simulink model "differential_steer"  (R2017b)
settings: Solver=FixedStepAuto  StartTime=0.0  StopTime=5  FixedStep=0.002  RelTol=1e-3
values from neighbouring files (symbols this model uses):
  B = 0.5    [main_differential_steer.m]
  input_type = 3    [main_bicycle.m]    (also in main_differential_steer.m; main_dynamic_bicycle.m)
  theta0 = 0    [main_differential_steer.m]    (also in main_dynamic_bicycle.m)
  x0 = 0    [main_differential_steer.m]    (also in main_dynamic_bicycle.m)
  y0 = 0    [main_differential_steer.m]    (also in main_dynamic_bicycle.m)
settings Model: Creator=zhenghe3  LastModifiedBy=zhenghe3

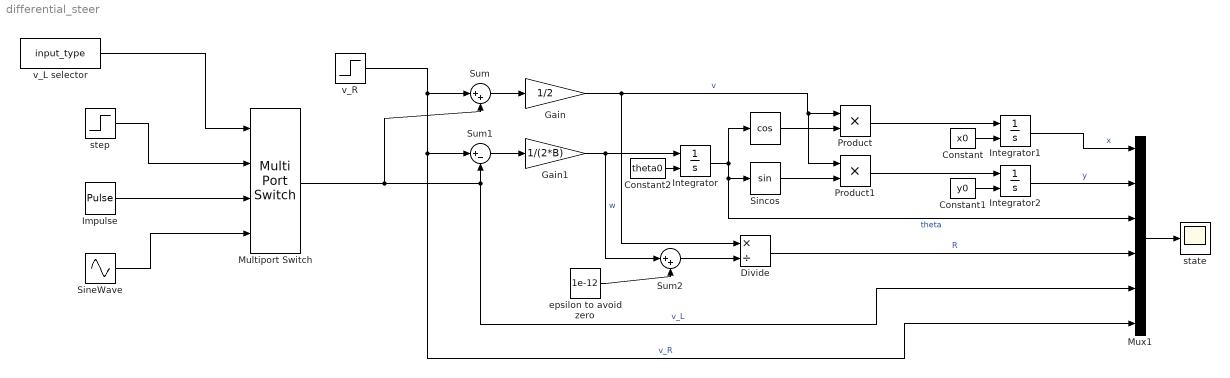
== system differential_steer ==
  " " : Trigonometry  Operator=cos
  Constant : Constant  Value=x0
  Constant1 : Constant  Value=y0
  Constant2 : Constant  Value=theta0
  Divide : Product  Inputs=*/
  Gain : Gain  Gain=1/2
  Gain1 : Gain  Gain=1/(2*B)
  Impulse : DiscretePulseGenerator  PulseType=Time based  Period=1  PulseWidth=50
  Integrator : Integrator  InitialConditionSource=external
  Integrator1 : Integrator  InitialConditionSource=external
  Integrator2 : Integrator  InitialConditionSource=external
  Multiport Switch : MultiPortSwitch
  Mux1 : Mux  Inputs=6
  Product : Product
  Product1 : Product
  Sincos : Trigonometry
  SineWave : Sin  Frequency=5  SampleTime=0
  Sum : Sum  Inputs=|++
  Sum1 : Sum  Inputs=|+-
  Sum2 : Sum  Inputs=|++
  epsilon to avoid zero : Constant  Value=1e-12
  state : Scope
  step : Step  Time=0  SampleTime=0
  v_L selector : Constant  Value=input_type
  v_R : Step  Time=0  After=1.5  SampleTime=0
  wires:
  v_R/1 -> Mux1/6, Sum1/1, Sum/1  "v_R"
  Multiport Switch/1 -> Mux1/5, Sum1/2, Sum/2  "v_L"
  Sum/1 -> Gain/1
  Gain/1 -> Product1/1, Product/1, Divide/1  "v"
  Sum1/1 -> Gain1/1
  Gain1/1 -> Integrator/1, Sum2/1  "w"
  Integrator/1 -> " "/1, Mux1/3, Sincos/1  "theta"
  " "/1 -> Product/2
  Sincos/1 -> Product1/2
  Product/1 -> Integrator1/1
  Product1/1 -> Integrator2/1
  Mux1/1 -> state/1
  Integrator1/1 -> Mux1/1  "x"
  Integrator2/1 -> Mux1/2  "y"
  v_L selector/1 -> Multiport Switch/1
  SineWave/1 -> Multiport Switch/4
  step/1 -> Multiport Switch/2
  Impulse/1 -> Multiport Switch/3
  epsilon to avoid zero/1 -> Sum2/2
  Sum2/1 -> Divide/2
  Constant/1 -> Integrator1/2
  Constant1/1 -> Integrator2/2
  Constant2/1 -> Integrator/2
  Divide/1 -> Mux1/4  "R"
